simulink model "Overtaking"  (R2024a)
settings: Solver=FixedStepDiscrete  StartTime=0.0  StopTime=inf  FixedStep=0.001  RelTol=1e-3  EnableMultiTasking=on
undefined symbols (not defined in the file): route1_frenet, route1_waypoint, route2_frenet, route2_waypoint, route3_frenet, route3_waypoint, route4_frenet, route4_waypoint, route5_frenet, route5_waypoint
libraries: CarMaker4SL x46, simulink x1, slpidlib x1
(part 2 of 3)

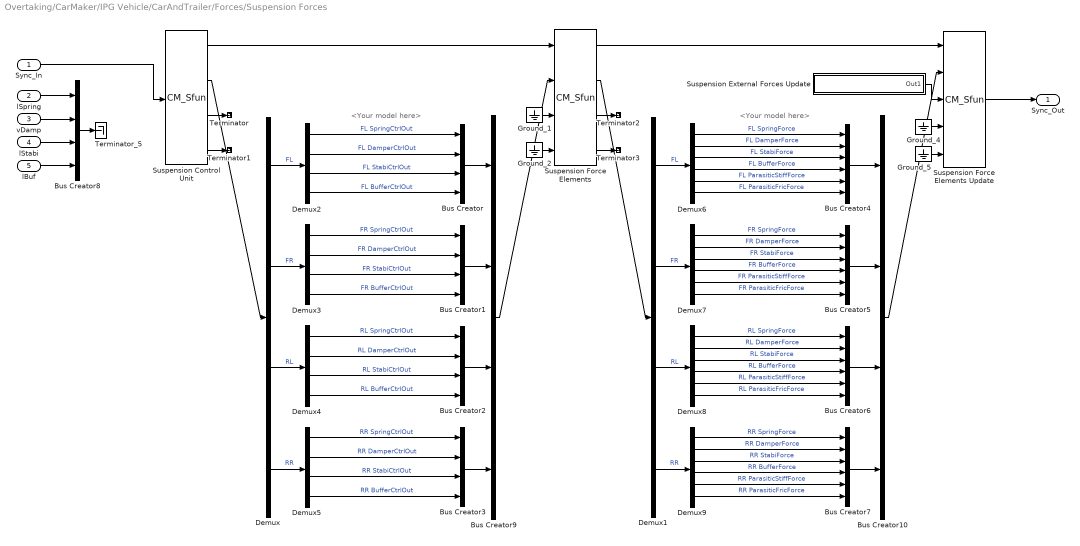
== system Overtaking/CarMaker/IPG Vehicle/CarAndTrailer/Forces/Suspension Forces ==
  note: <Your model here>
  note: <Your model here>
  Sync_In : Inport
  lSpring : Inport  Port=2
  vDamp : Inport  Port=3
  lStabi : Inport  Port=4
  lBuf : Inport  Port=5
  Bus Creator{,1..3,8..10} (7 alike) : BusCreator  Inputs=4
  Bus Creator{4..7} (4 alike) : BusCreator  Inputs=6
  Demux{,1..5} (6 alike) : Demux
  Demux{6..9} (4 alike) : Demux  Outputs=6
  Ground_{1..2,4..5} (4 alike) : Ground
  Suspension Control Unit : S-Function  FunctionName=CM_Sfun  Parameters='ForcesSuspControl'  SFunctionDeploymentMode=off  EnableBusSupport=off
  Suspension External Forces Update : Subsystem
  Suspension Force Elements : S-Function  FunctionName=CM_Sfun  Parameters='ForcesSusp'  SFunctionDeploymentMode=off  EnableBusSupport=off
  Suspension Force Elements Update : S-Function  FunctionName=CM_Sfun  Parameters='ForcesSuspUpd'  SFunctionDeploymentMode=off  EnableBusSupport=off
  Terminator{,1..3} (4 alike) : Terminator
  Terminator_5 : Terminator
  Sync_Out : Outport  VectorParamsAs1DForOutWhenUnconnected=off
  wires:
  vDamp/1 -> Bus Creator8/2
  lStabi/1 -> Bus Creator8/3
  lBuf/1 -> Bus Creator8/4
  lSpring/1 -> Bus Creator8/1
  Bus Creator4/1 -> Bus Creator10/1
  Bus Creator5/1 -> Bus Creator10/2
  Bus Creator6/1 -> Bus Creator10/3
  Bus Creator7/1 -> Bus Creator10/4
  Demux6/1 -> Bus Creator4/1  "FL SpringForce"
  Demux9/1 -> Bus Creator7/1  "RR SpringForce"
  Demux9/2 -> Bus Creator7/2  "RR DamperForce"
  Demux9/3 -> Bus Creator7/3  "RR StabiForce"
  Demux9/4 -> Bus Creator7/4  "RR BufferForce"
  Demux9/5 -> Bus Creator7/5  "RR ParasiticStiffForce"
  Demux9/6 -> Bus Creator7/6  "RR ParasiticFricForce"
  Demux8/1 -> Bus Creator6/1  "RL SpringForce"
  Demux8/2 -> Bus Creator6/2  "RL DamperForce"
  Demux8/4 -> Bus Creator6/4  "RL BufferForce"
  Demux8/5 -> Bus Creator6/5  "RL ParasiticStiffForce"
  Demux8/6 -> Bus Creator6/6  "RL ParasiticFricForce"
  Demux8/3 -> Bus Creator6/3  "RL StabiForce"
  Demux7/1 -> Bus Creator5/1  "FR SpringForce"
  Demux7/2 -> Bus Creator5/2  "FR DamperForce"
  Demux7/3 -> Bus Creator5/3  "FR StabiForce"
  Demux7/4 -> Bus Creator5/4  "FR BufferForce"
  Demux7/5 -> Bus Creator5/5  "FR ParasiticStiffForce"
  Demux7/6 -> Bus Creator5/6  "FR ParasiticFricForce"
  Demux6/2 -> Bus Creator4/2  "FL DamperForce"
  Demux6/3 -> Bus Creator4/3  "FL StabiForce"
  Demux6/4 -> Bus Creator4/4  "FL BufferForce"
  Demux6/5 -> Bus Creator4/5  "FL ParasiticStiffForce"
  Demux6/6 -> Bus Creator4/6  "FL ParasiticFricForce"
  Demux/1 -> Demux2/1  "FL"
  Bus Creator1/1 -> Bus Creator9/2
  Demux/2 -> Demux3/1  "FR"
  Bus Creator2/1 -> Bus Creator9/3
  Demux/3 -> Demux4/1  "RL"
  Bus Creator3/1 -> Bus Creator9/4
  Demux2/1 -> Bus Creator/1  "FL SpringCtrlOut"
  Demux/4 -> Demux5/1  "RR"
  Demux5/1 -> Bus Creator3/1  "RR SpringCtrlOut"
  Demux5/2 -> Bus Creator3/2  "RR DamperCtrlOut"
  Demux5/3 -> Bus Creator3/3  "RR StabiCtrlOut"
  Demux5/4 -> Bus Creator3/4  "RR BufferCtrlOut"
  Demux4/1 -> Bus Creator2/1  "RL SpringCtrlOut"
  Demux4/2 -> Bus Creator2/2  "RL DamperCtrlOut"
  Demux4/4 -> Bus Creator2/4  "RL BufferCtrlOut"
  Demux4/3 -> Bus Creator2/3  "RL StabiCtrlOut"
  Demux3/1 -> Bus Creator1/1  "FR SpringCtrlOut"
  Demux3/2 -> Bus Creator1/2  "FR DamperCtrlOut"
  Demux3/3 -> Bus Creator1/3  "FR StabiCtrlOut"
  Demux3/4 -> Bus Creator1/4  "FR BufferCtrlOut"
  Demux2/2 -> Bus Creator/2  "FL DamperCtrlOut"
  Demux2/3 -> Bus Creator/3  "FL StabiCtrlOut"
  Demux2/4 -> Bus Creator/4  "FL BufferCtrlOut"
  Bus Creator/1 -> Bus Creator9/1
  Demux1/1 -> Demux6/1  "FL"
  Demux1/2 -> Demux7/1  "FR"
  Demux1/3 -> Demux8/1  "RL"
  Demux1/4 -> Demux9/1  "RR"
  Suspension Control Unit/2 -> Demux/1
  Suspension Control Unit/3 -> Terminator/1
  Suspension Control Unit/4 -> Terminator1/1
  Sync_In/1 -> Suspension Control Unit/1
  Suspension Force Elements/2 -> Demux1/1
  Suspension Force Elements/3 -> Terminator2/1
  Suspension Force Elements/4 -> Terminator3/1
  Suspension Control Unit/1 -> Suspension Force Elements/1
  Bus Creator9/1 -> Suspension Force Elements/2
  Bus Creator8/1 -> Terminator_5/1
  Ground_1/1 -> Suspension Force Elements/3
  Ground_2/1 -> Suspension Force Elements/4
  Suspension Force Elements Update/1 -> Sync_Out/1
  Suspension Force Elements/1 -> Suspension Force Elements Update/1
  Bus Creator10/1 -> Suspension Force Elements Update/2
  Ground_4/1 -> Suspension Force Elements Update/4
  Ground_5/1 -> Suspension Force Elements Update/5
  Suspension External Forces Update/1(Out1) -> Suspension Force Elements Update/3

== system Overtaking/CarMaker/IPG Vehicle/CarAndTrailer/Forces/Tires ==
  note: The TireXX_Out signals will only be used if FileIdent is "CarMaker-Tire-CM4SL" in the tire parameter file!
      | An example parameter file can be found in Data/Tire/DT_CM4SL_UserTire.
  Sync_In : Inport
  TireFL_In : Inport  Port=2
  TireFR_In : Inport  Port=3
  TireRL_In : Inport  Port=4
  TireRR_In : Inport  Port=5
  Bus Creator{1..4} (4 alike) : BusCreator  Inputs=11
  Demux{1..3,8} (4 alike) : Demux  Outputs=7
      settings: DisplayOption=none
  TireFL : Subsystem
  TireFR : Subsystem
  TireRL : Subsystem
  TireRR : Subsystem
  TireFL_Out : Outport  VectorParamsAs1DForOutWhenUnconnected=off
  TireFR_Out : Outport  Port=2  VectorParamsAs1DForOutWhenUnconnected=off
  TireRL_Out : Outport  Port=3  VectorParamsAs1DForOutWhenUnconnected=off
  TireRR_Out : Outport  Port=4  VectorParamsAs1DForOutWhenUnconnected=off
  wires:
  Sync_In/1 -> TireRR/1(Sync_In), TireRL/1(Sync_In), TireFR/1(Sync_In), TireFL/1(Sync_In)
  Bus Creator4/1 -> TireRR_Out/1
  Bus Creator2/1 -> TireRL_Out/1
  Bus Creator1/1 -> TireFR_Out/1
  Demux3/5 -> TireRR/6(Rim_turnv)  "Tire_In Rim_turnv"
  Demux3/4 -> TireRR/5(Rim_rotv)  "Tire_In Rim_rotv"
  Demux3/1 -> TireRR/2(Load)  "Tire_In Load"
  Demux3/7 -> TireRR/8(muRoad)  "Tire_In mu"
  Demux3/6 -> TireRR/7(InclinAngle)  "Tire_In Camber"
  Demux3/2 -> TireRR/3(vxtrans)  "Tire_In vxtrans"
  Demux3/3 -> TireRR/4(vytrans)  "Tire_In vytrans"
  TireRR/11(AlignTrq) -> Bus Creator4/11  "Tire_Out AlignTrq"
  TireRR/10(RollResist) -> Bus Creator4/10  "Tire_Out RollResist"
  TireRR/9(OverturnTrq) -> Bus Creator4/9  "Tire_Out OverturnTrq"
  TireRR/8(LoadFrc) -> Bus Creator4/8  "Tire_Out LoadFrc"
  TireRR/7(SideFrc) -> Bus Creator4/7  "Tire_Out SideFrc"
  TireRR/6(LongFrc) -> Bus Creator4/6  "Tire_Out LongFrc"
  TireRR/5(vBelt) -> Bus Creator4/5  "Tire_Out vBelt"
  TireRR/4(rBelt_eff) -> Bus Creator4/4  "Tire_Out rBelt_eff"
  TireRR/3(TurnSlp) -> Bus Creator4/3  "Tire_Out TurnSlp"
  TireRR/1(Slp) -> Bus Creator4/1  "Tire_Out Slp"
  TireRR/2(Alpha) -> Bus Creator4/2  "Tire_Out Alpha"
  Demux2/5 -> TireRL/6(Rim_turnv)  "Tire_In Rim_turnv"
  Demux2/4 -> TireRL/5(Rim_rotv)  "Tire_In Rim_rotv"
  Demux2/1 -> TireRL/2(Load)  "Tire_In Load"
  Demux2/7 -> TireRL/8(muRoad)  "Tire_In mu"
  Demux2/6 -> TireRL/7(InclinAngle)  "Tire_In Camber"
  Demux2/2 -> TireRL/3(vxtrans)  "Tire_In vxtrans"
  Demux2/3 -> TireRL/4(vytrans)  "Tire_In vytrans"
  TireRL/11(AlignTrq) -> Bus Creator2/11  "Tire_Out AlignTrq"
  TireRL/10(RollResist) -> Bus Creator2/10  "Tire_Out RollResist"
  TireRL/9(OverturnTrq) -> Bus Creator2/9  "Tire_Out OverturnTrq"
  TireRL/8(LoadFrc) -> Bus Creator2/8  "Tire_Out LoadFrc"
  TireRL/7(SideFrc) -> Bus Creator2/7  "Tire_Out SideFrc"
  TireRL/6(LongFrc) -> Bus Creator2/6  "Tire_Out LongFrc"
  TireRL/5(vBelt) -> Bus Creator2/5  "Tire_Out vBelt"
  TireRL/4(rBelt_eff) -> Bus Creator2/4  "Tire_Out rBelt_eff"
  TireRL/3(TurnSlp) -> Bus Creator2/3  "Tire_Out TurnSlp"
  TireRL/1(Slp) -> Bus Creator2/1  "Tire_Out Slp"
  TireRL/2(Alpha) -> Bus Creator2/2  "Tire_Out Alpha"
  Demux1/5 -> TireFR/6(Rim_turnv)  "Tire_In Rim_turnv"
  Demux1/4 -> TireFR/5(Rim_rotv)  "Tire_In Rim_rotv"
  Demux1/1 -> TireFR/2(Load)  "Tire_In Load"
  Demux1/7 -> TireFR/8(muRoad)  "Tire_In mu"
  Demux1/6 -> TireFR/7(InclinAngle)  "Tire_In Camber"
  Demux1/2 -> TireFR/3(vxtrans)  "Tire_In vxtrans"
  Demux1/3 -> TireFR/4(vytrans)  "Tire_In vytrans"
  TireFR/11(AlignTrq) -> Bus Creator1/11  "Tire_Out AlignTrq"
  TireFR/10(RollResist) -> Bus Creator1/10  "Tire_Out RollResist"
  TireFR/9(OverturnTrq) -> Bus Creator1/9  "Tire_Out OverturnTrq"
  TireFR/8(LoadFrc) -> Bus Creator1/8  "Tire_Out LoadFrc"
  TireFR/7(SideFrc) -> Bus Creator1/7  "Tire_Out SideFrc"
  TireFR/6(LongFrc) -> Bus Creator1/6  "Tire_Out LongFrc"
  TireFR/5(vBelt) -> Bus Creator1/5  "Tire_Out vBelt"
  TireFR/4(rBelt_eff) -> Bus Creator1/4  "Tire_Out rBelt_eff"
  TireFR/3(TurnSlp) -> Bus Creator1/3  "Tire_Out TurnSlp"
  TireFR/1(Slp) -> Bus Creator1/1  "Tire_Out Slp"
  TireFR/2(Alpha) -> Bus Creator1/2  "Tire_Out Alpha"
  Demux8/5 -> TireFL/6(Rim_turnv)  "Tire_In Rim_turnv"
  Demux8/4 -> TireFL/5(Rim_rotv)  "Tire_In Rim_rotv"
  TireFL_In/1 -> Demux8/1
  Demux8/1 -> TireFL/2(Load)  "Tire_In Load"
  Demux8/7 -> TireFL/8(muRoad)  "Tire_In mu"
  Demux8/6 -> TireFL/7(InclinAngle)  "Tire_In Camber"
  Demux8/2 -> TireFL/3(vxtrans)  "Tire_In vxtrans"
  Demux8/3 -> TireFL/4(vytrans)  "Tire_In vytrans"
  TireFL/11(AlignTrq) -> Bus Creator3/11  "Tire_Out AlignTrq"
  TireFL/10(RollResist) -> Bus Creator3/10  "Tire_Out RollResist"
  TireFL/9(OverturnTrq) -> Bus Creator3/9  "Tire_Out OverturnTrq"
  TireFL/8(LoadFrc) -> Bus Creator3/8  "Tire_Out LoadFrc"
  TireFL/7(SideFrc) -> Bus Creator3/7  "Tire_Out SideFrc"
  TireFL/6(LongFrc) -> Bus Creator3/6  "Tire_Out LongFrc"
  TireFL/5(vBelt) -> Bus Creator3/5  "Tire_Out vBelt"
  TireFL/4(rBelt_eff) -> Bus Creator3/4  "Tire_Out rBelt_eff"
  TireFL/3(TurnSlp) -> Bus Creator3/3  "Tire_Out TurnSlp"
  TireFL/1(Slp) -> Bus Creator3/1  "Tire_Out Slp"
  TireFL/2(Alpha) -> Bus Creator3/2  "Tire_Out Alpha"
  Bus Creator3/1 -> TireFL_Out/1
  TireFR_In/1 -> Demux1/1
  TireRL_In/1 -> Demux2/1
  TireRR_In/1 -> Demux3/1

== system Overtaking/CarMaker/IPG Vehicle/CarAndTrailer/Forces/Vehicle Forces ==
  Sync_In : Inport
  Bus Creator1 : BusCreator  Inputs=12
  Bus Creator8 : BusCreator  Inputs=16
  BusCreator1 : BusCreator  Inputs=4
  BusCreator2 : BusCreator  Inputs=9
  Demux : Demux  Outputs=16
      settings: DisplayOption=none
  Demux1 : Demux  Outputs=12
      settings: DisplayOption=none
  Demux2 : Demux  Outputs=13
      settings: DisplayOption=none
  Forces : S-Function  FunctionName=CM_Sfun  Parameters='Forces'  SFunctionDeploymentMode=off  EnableBusSupport=off
  Terminator : Terminator
  Sync_Out : Outport  VectorParamsAs1DForOutWhenUnconnected=off
  Car.Virtual : Outport  Port=2  VectorParamsAs1DForOutWhenUnconnected=off
  Car.Aero : Outport  Port=3  VectorParamsAs1DForOutWhenUnconnected=off
  Car.Load : Outport  Port=4  VectorParamsAs1DForOutWhenUnconnected=off
  wires:
  BusCreator1/1 -> Terminator/1  "Aero IF (in)"
  Demux2/13 -> BusCreator2/9  "car Aero Trq_1 z"
  Demux2/12 -> BusCreator2/8  "car Aero Trq_1 y"
  Demux2/11 -> BusCreator2/7  "car Aero Trq_1 x"
  Demux2/10 -> BusCreator2/6  "car Aero Frc_1 z"
  Demux2/9 -> BusCreator2/5  "car Aero Frc_1 y"
  Demux2/8 -> BusCreator2/4  "car Aero Frc_1 x"
  Demux2/7 -> BusCreator2/3  "car Aero PoA_1 z"
  Demux2/6 -> BusCreator2/2  "car Aero PoA_1 y"
  Demux2/5 -> BusCreator2/1  "car Aero PoA_1 x"
  Demux2/4 -> BusCreator1/4  "car Aero tau_1"
  Demux2/3 -> BusCreator1/3  "car Aero ApproachVel_1 z"
  Demux2/2 -> BusCreator1/2  "car Aero ApproachVel_1 y"
  Demux2/1 -> BusCreator1/1  "car Aero ApproachVel_1 x"
  Demux/16 -> Bus Creator8/16  "Car Load_3 tz"
  Demux/15 -> Bus Creator8/15  "Car Load_3 ty"
  Demux/14 -> Bus Creator8/14  "Car Load_3 tx"
  Demux/13 -> Bus Creator8/13  "Car Load_3 mass"
  Demux1/12 -> Bus Creator1/12  "Car Virtual Trq_0 z"
  Demux1/11 -> Bus Creator1/11  "Car Virtual Trq_0 y"
  Demux1/10 -> Bus Creator1/10  "Car Virtual Trq_0 x"
  Demux1/9 -> Bus Creator1/9  "Car Virtual Trq_1 z"
  Demux1/8 -> Bus Creator1/8  "Car Virtual Trq_1 y"
  Demux1/7 -> Bus Creator1/7  "Car Virtual Trq_1 x"
  Demux1/6 -> Bus Creator1/6  "Car Virtual Frc_0 z"
  Demux1/5 -> Bus Creator1/5  "Car Virtual Frc_0 y"
  Demux1/4 -> Bus Creator1/4  "Car Virtual Frc_0 x"
  Sync_In/1 -> Forces/1
  Forces/1 -> Sync_Out/1
  BusCreator2/1 -> Car.Aero/1
  Demux1/1 -> Bus Creator1/1  "Car Virtual Frc_1 x"
  Demux1/2 -> Bus Creator1/2  "Car Virtual Frc_1 y"
  Demux1/3 -> Bus Creator1/3  "Car Virtual Frc_1 z"
  Forces/3 -> Demux2/1
  Forces/2 -> Demux1/1
  Bus Creator1/1 -> Car.Virtual/1
  Bus Creator8/1 -> Car.Load/1
  Demux/1 -> Bus Creator8/1  "Car Load_0 mass"
  Demux/2 -> Bus Creator8/2  "Car Load_0 tx"
  Demux/3 -> Bus Creator8/3  "Car Load_0 ty"
  Demux/4 -> Bus Creator8/4  "Car Load_0 tz"
  Demux/5 -> Bus Creator8/5  "Car Load_1 mass"
  Demux/6 -> Bus Creator8/6  "Car Load_1 tx"
  Demux/7 -> Bus Creator8/7  "Car Load_1 ty"
  Demux/8 -> Bus Creator8/8  "Car Load_1 tz"
  Demux/9 -> Bus Creator8/9  "Car Load_2 mass"
  Demux/10 -> Bus Creator8/10  "Car Load_2 tx"
  Demux/11 -> Bus Creator8/11  "Car Load_2 ty"
  Demux/12 -> Bus Creator8/12  "Car Load_2 tz"
  Forces/4 -> Demux/1

== system Overtaking/CarMaker/IPG Vehicle/CarAndTrailer/Trailer/CreateBus Car.Hitch.FrcTrq ==
  In1 : Inport
  Bus Creator7 : BusCreator  Inputs=6
  Demux7 : Demux  Outputs=6
      settings: DisplayOption=none
  Out1 : Outport  VectorParamsAs1DForOutWhenUnconnected=off
  wires:
  In1/1 -> Demux7/1
  Bus Creator7/1 -> Out1/1
  Demux7/6 -> Bus Creator7/6  "Car Hitch Trq2Car z"
  Demux7/5 -> Bus Creator7/5  "Car Hitch Trq2Car y"
  Demux7/4 -> Bus Creator7/4  "Car Hitch Trq2Car x"
  Demux7/3 -> Bus Creator7/3  "Car Hitch Frc2Car z"
  Demux7/2 -> Bus Creator7/2  "Car Hitch Frc2Car y"
  Demux7/1 -> Bus Creator7/1  "Car Hitch Frc2Car x"

== system Overtaking/CarMaker/IPG Vehicle/CarAndTrailer/Trailer/CreateBus Vhcl.Motion ==
  In1 : Inport
  BusCreator : BusCreator  Inputs=15
  Demux : Demux  Outputs=15
      settings: DisplayOption=none
  Out1 : Outport  VectorParamsAs1DForOutWhenUnconnected=off
  wires:
  Demux/15 -> BusCreator/15  "Vhcl YawAcc"
  Demux/14 -> BusCreator/14  "Vhcl YawVel"
  Demux/13 -> BusCreator/13  "Vhcl Yaw"
  Demux/12 -> BusCreator/12  "Vhcl PitchAcc"
  Demux/11 -> BusCreator/11  "Vhcl PitchVel"
  Demux/10 -> BusCreator/10  "Vhcl Pitch"
  Demux/9 -> BusCreator/9  "Vhcl RollAcc"
  Demux/8 -> BusCreator/8  "Vhcl RollVel"
  Demux/7 -> BusCreator/7  "Vhcl Roll"
  Demux/6 -> BusCreator/6  "Vhcl Hitch_Pos z"
  Demux/5 -> BusCreator/5  "Vhcl Hitch_Pos y"
  Demux/4 -> BusCreator/4  "Vhcl Hitch_Pos x"
  Demux/3 -> BusCreator/3  "Vhcl sRoad"
  Demux/2 -> BusCreator/2  "Vhcl Distance"
  Demux/1 -> BusCreator/1  "Vhcl v"
  In1/1 -> Demux/1
  BusCreator/1 -> Out1/1

== system Overtaking/CarMaker/IPG Vehicle/CarAndTrailer/Trailer/CreateBus Vhcl.PoI ==
  In1 : Inport
  Bus Creator3 : BusCreator  Inputs=18
  Demux3 : Demux  Outputs=18
      settings: DisplayOption=none
  Out1 : Outport  VectorParamsAs1DForOutWhenUnconnected=off
  wires:
  Demux3/18 -> Bus Creator3/18  "Vhcl PoI_GCS Elev"
  Demux3/17 -> Bus Creator3/17  "Vhcl PoI_GCS Lat"
  Demux3/16 -> Bus Creator3/16  "Vhcl PoI_GCS Long"
  Demux3/15 -> Bus Creator3/15  "Vhcl PoI_Acc_1 z"
  Demux3/14 -> Bus Creator3/14  "Vhcl PoI_Acc_1 y"
  Demux3/13 -> Bus Creator3/13  "Vhcl PoI_Acc_1 x"
  Demux3/12 -> Bus Creator3/12  "Vhcl PoI_Vel_1 z"
  Demux3/11 -> Bus Creator3/11  "Vhcl PoI_Vel_1 y"
  Demux3/10 -> Bus Creator3/10  "Vhcl PoI_Vel_1 x"
  Demux3/9 -> Bus Creator3/9  "Vhcl PoI_Acc z"
  Demux3/8 -> Bus Creator3/8  "Vhcl PoI_Acc y"
  Demux3/7 -> Bus Creator3/7  "Vhcl PoI_Acc x"
  Demux3/6 -> Bus Creator3/6  "Vhcl PoI_Vel z"
  Demux3/5 -> Bus Creator3/5  "Vhcl PoI_Vel y"
  Demux3/4 -> Bus Creator3/4  "Vhcl PoI_Vel x"
  Demux3/3 -> Bus Creator3/3  "Vhcl PoI_Pos z"
  Demux3/2 -> Bus Creator3/2  "Vhcl PoI_Pos y"
  In1/1 -> Demux3/1
  Bus Creator3/1 -> Out1/1
  Demux3/1 -> Bus Creator3/1  "Vhcl PoI_Pos x"

== system Overtaking/CarMaker/IPG Vehicle/CarAndTrailer/Trailer/CreateBus Vhcl.Steering ==
  In1 : Inport
  Bus Creator3 : BusCreator  Inputs=4
  Demux : Demux
      settings: DisplayOption=none
  Out1 : Outport  VectorParamsAs1DForOutWhenUnconnected=off
  wires:
  Bus Creator3/1 -> Out1/1
  Demux/1 -> Bus Creator3/1  "Vhcl Steering Ang"
  Demux/3 -> Bus Creator3/3  "Vhcl Steering AngAcc"
  Demux/2 -> Bus Creator3/2  "Vhcl Steering AngVel"
  Demux/4 -> Bus Creator3/4  "Vhcl Steering Trq"
  In1/1 -> Demux/1

== system Overtaking/CarMaker/IPG Vehicle/CarAndTrailer/Trailer/CreateBus Vhcl.Wheel.FL ==
  In1 : Inport
  Bus Creator3 : BusCreator  Inputs=14
  Demux3 : Demux  Outputs=14
      settings: DisplayOption=none
  Out1 : Outport  VectorParamsAs1DForOutWhenUnconnected=off
  wires:
  Demux3/14 -> Bus Creator3/14  "Vhcl Wheel FL Trq_WhlBearing"
  Demux3/13 -> Bus Creator3/13  "Vhcl Wheel FL Trq_T2W"
  Demux3/12 -> Bus Creator3/12  "Vhcl Wheel FL SideSlip"
  Demux3/11 -> Bus Creator3/11  "Vhcl Wheel FL LongSlip"
  Demux3/10 -> Bus Creator3/10  "Vhcl Wheel FL vBelt"
  Demux3/9 -> Bus Creator3/9  "Vhcl Wheel FL Fz"
  Demux3/8 -> Bus Creator3/8  "Vhcl Wheel FL Fy"
  Demux3/7 -> Bus Creator3/7  "Vhcl Wheel FL Fx"
  Demux3/6 -> Bus Creator3/6  "Vhcl Wheel FL r_zxy z"
  Demux3/5 -> Bus Creator3/5  "Vhcl Wheel FL r_zxy y"
  Demux3/4 -> Bus Creator3/4  "Vhcl Wheel FL r_zxy x"
  Demux3/3 -> Bus Creator3/3  "Vhcl Wheel FL t z"
  Demux3/2 -> Bus Creator3/2  "Vhcl Wheel FL t y"
  In1/1 -> Demux3/1
  Bus Creator3/1 -> Out1/1
  Demux3/1 -> Bus Creator3/1  "Vhcl Wheel FL t x"

== system Overtaking/CarMaker/IPG Vehicle/CarAndTrailer/Trailer/CreateBus Vhcl.Wheel.FR ==
  In1 : Inport
  Bus Creator3 : BusCreator  Inputs=14
  Demux3 : Demux  Outputs=14
      settings: DisplayOption=none
  Out1 : Outport  VectorParamsAs1DForOutWhenUnconnected=off
  wires:
  Demux3/14 -> Bus Creator3/14  "Vhcl Wheel FR Trq_WhlBearing"
  Demux3/13 -> Bus Creator3/13  "Vhcl Wheel FR Trq_T2W"
  Demux3/12 -> Bus Creator3/12  "Vhcl Wheel FR SideSlip"
  Demux3/11 -> Bus Creator3/11  "Vhcl Wheel FR LongSlip"
  Demux3/10 -> Bus Creator3/10  "Vhcl Wheel FR vBelt"
  Demux3/9 -> Bus Creator3/9  "Vhcl Wheel FR Fz"
  Demux3/8 -> Bus Creator3/8  "Vhcl Wheel FR Fy"
  Demux3/7 -> Bus Creator3/7  "Vhcl Wheel FR Fx"
  Demux3/6 -> Bus Creator3/6  "Vhcl Wheel FR r_zxy z"
  Demux3/5 -> Bus Creator3/5  "Vhcl Wheel FR r_zxy y"
  Demux3/4 -> Bus Creator3/4  "Vhcl Wheel FR r_zxy x"
  Demux3/3 -> Bus Creator3/3  "Vhcl Wheel FR t z"
  Demux3/2 -> Bus Creator3/2  "Vhcl Wheel FR t y"
  In1/1 -> Demux3/1
  Bus Creator3/1 -> Out1/1
  Demux3/1 -> Bus Creator3/1  "Vhcl Wheel FR t x"

== system Overtaking/CarMaker/IPG Vehicle/CarAndTrailer/Trailer/CreateBus Vhcl.Wheel.RL ==
  In1 : Inport
  Bus Creator3 : BusCreator  Inputs=14
  Demux3 : Demux  Outputs=14
      settings: DisplayOption=none
  Out1 : Outport  VectorParamsAs1DForOutWhenUnconnected=off
  wires:
  Demux3/14 -> Bus Creator3/14  "Vhcl Wheel RL Trq_WhlBearing"
  Demux3/13 -> Bus Creator3/13  "Vhcl Wheel RL Trq_T2W"
  Demux3/12 -> Bus Creator3/12  "Vhcl Wheel RL SideSlip"
  Demux3/11 -> Bus Creator3/11  "Vhcl Wheel RL LongSlip"
  Demux3/10 -> Bus Creator3/10  "Vhcl Wheel RL vBelt"
  Demux3/9 -> Bus Creator3/9  "Vhcl Wheel RL Fz"
  Demux3/8 -> Bus Creator3/8  "Vhcl Wheel RL Fy"
  Demux3/7 -> Bus Creator3/7  "Vhcl Wheel RL Fx"
  Demux3/6 -> Bus Creator3/6  "Vhcl Wheel RL r_zxy z"
  Demux3/5 -> Bus Creator3/5  "Vhcl Wheel RL r_zxy y"
  Demux3/4 -> Bus Creator3/4  "Vhcl Wheel RL r_zxy x"
  Demux3/3 -> Bus Creator3/3  "Vhcl Wheel RL t z"
  Demux3/2 -> Bus Creator3/2  "Vhcl Wheel RL t y"
  In1/1 -> Demux3/1
  Bus Creator3/1 -> Out1/1
  Demux3/1 -> Bus Creator3/1  "Vhcl Wheel RL t x"

== system Overtaking/CarMaker/IPG Vehicle/CarAndTrailer/Trailer/CreateBus Vhcl.Wheel.RR ==
  In1 : Inport
  Bus Creator3 : BusCreator  Inputs=14
  Demux3 : Demux  Outputs=14
      settings: DisplayOption=none
  Out1 : Outport  VectorParamsAs1DForOutWhenUnconnected=off
  wires:
  Demux3/14 -> Bus Creator3/14  "Vhcl Wheel RR Trq_WhlBearing"
  Demux3/13 -> Bus Creator3/13  "Vhcl Wheel RR Trq_T2W"
  Demux3/12 -> Bus Creator3/12  "Vhcl Wheel RR SideSlip"
  Demux3/11 -> Bus Creator3/11  "Vhcl Wheel RR LongSlip"
  Demux3/10 -> Bus Creator3/10  "Vhcl Wheel RR vBelt"
  Demux3/9 -> Bus Creator3/9  "Vhcl Wheel RR Fz"
  Demux3/8 -> Bus Creator3/8  "Vhcl Wheel RR Fy"
  Demux3/7 -> Bus Creator3/7  "Vhcl Wheel RR Fx"
  Demux3/6 -> Bus Creator3/6  "Vhcl Wheel RR r_zxy z"
  Demux3/5 -> Bus Creator3/5  "Vhcl Wheel RR r_zxy y"
  Demux3/4 -> Bus Creator3/4  "Vhcl Wheel RR r_zxy x"
  Demux3/3 -> Bus Creator3/3  "Vhcl Wheel RR t z"
  Demux3/2 -> Bus Creator3/2  "Vhcl Wheel RR t y"
  In1/1 -> Demux3/1
  Bus Creator3/1 -> Out1/1
  Demux3/1 -> Bus Creator3/1  "Vhcl Wheel RR t x"

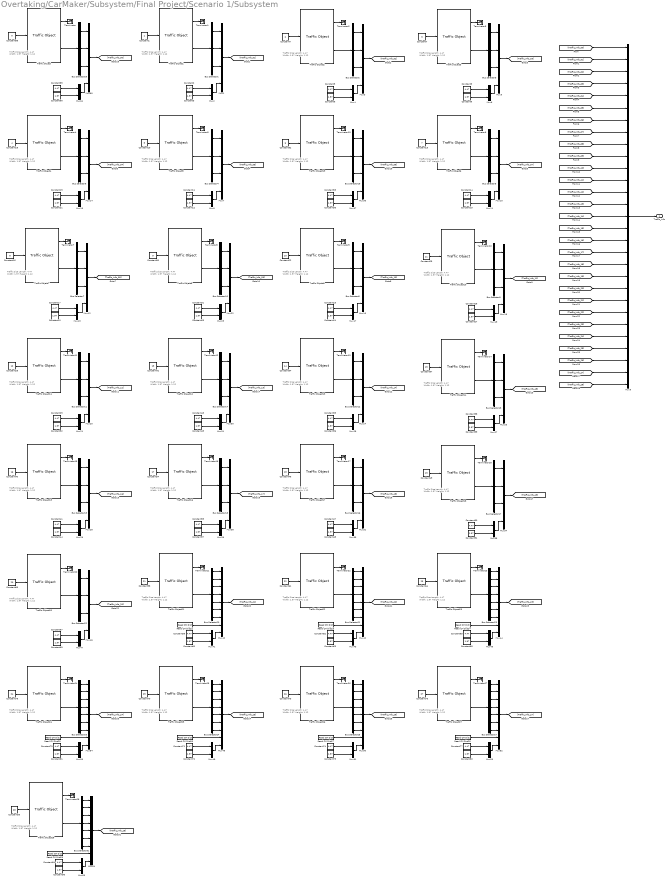
== system Overtaking/CarMaker/Subsystem/Final Project/Scenario 1/Subsystem ==
  note: Traffic Size
      | Length: 4.47
      | Width: 1.97
      | Height: 1.12
  note: Traffic Size
      | Length: 4.47
      | Width: 1.97
      | Height: 1.12
  note: Traffic Size
      | Length: 4.47
      | Width: 1.97
      | Height: 1.12
  note: Traffic Size
      | Length: 4.47
      | Width: 1.97
      | Height: 1.12
  note: Traffic Size
      | Length: 4.47
      | Width: 1.97
      | Height: 1.12
  note: Traffic Size
      | Length: 4.47
      | Width: 1.97
      | Height: 1.12
  note: Traffic Size
      | Length: 4.47
      | Width: 1.97
      | Height: 1.12
  note: Traffic Size
      | Length: 4.47
      | Width: 1.97
      | Height: 1.12
  note: Traffic Size
      | Length: 4.47
      | Width: 1.97
      | Height: 1.12
  note: Traffic Size
      | Length: 4.47
      | Width: 1.97
      | Height: 1.12
  note: Traffic Size
      | Length: 4.47
      | Width: 1.97
      | Height: 1.12
  note: Traffic Size
      | Length: 4.47
      | Width: 1.97
      | Height: 1.12
  note: Traffic Size
      | Length: 4.47
      | Width: 1.97
      | Height: 1.12
  note: Traffic Size
      | Length: 4.47
      | Width: 1.97
      | Height: 1.12
  note: Traffic Size
      | Length: 4.47
      | Width: 1.97
      | Height: 1.12
  note: Traffic Size
      | Length: 4.47
      | Width: 1.97
      | Height: 1.12
  note: Traffic Size
      | Length: 4.47
      | Width: 1.97
      | Height: 1.12
  note: Traffic Size
      | Length: 4.47
      | Width: 1.97
      | Height: 1.12
  note: Traffic Size
      | Length: 4.47
      | Width: 1.97
      | Height: 1.12
  note: Traffic Size
      | Length: 4.47
      | Width: 1.97
      | Height: 1.12
  note: Traffic Size
      | Length: 4.47
      | Width: 1.97
      | Height: 1.12
  note: Traffic Size
      | Length: 4.47
      | Width: 1.97
      | Height: 1.12
  note: Traffic Size
      | Length: 4.47
      | Width: 1.97
      | Height: 1.12
  note: Traffic Size
      | Length: 4.47
      | Width: 1.97
      | Height: 1.12
  note: Traffic Size
      | Length: 4.47
      | Width: 1.97
      | Height: 1.12
  note: Traffic Size
      | Length: 4.47
      | Width: 1.97
      | Height: 1.12
  note: Traffic Size
      | Length: 4.47
      | Width: 1.97
      | Height: 1.12
  note: Traffic Size
      | Length: 4.47
      | Width: 1.97
      | Height: 1.12
  note: Traffic Size
      | Length: 4.47
      | Width: 1.97
      | Height: 1.12
  Bus Selector{1..19,22,29} (21 alike) : BusSelector  OutputSignals=t_0 x,t_0 y,r_zyx z
  Bus Selector{20..21,23..27,31} (8 alike) : BusSelector  OutputSignals=t_0 x,t_0 y,v_0 x,v_0 y,a_0 x,a_0 y,r_zyx z
  Constant1 : Constant
  Constant10 : Constant  Value=5
  Constant{2,5,8,11,14,17,19,23,26,29,31,35,38,41,43,47,50,53,55,59,62,65,67,71,74,77,79,89,94} (29 alike) : Constant  Value=4.47
  Constant{3,6,9,12,15,20..21,24,27,32..33,36,39,44..45,48,51,56..57,60,63,68..69,72,75,80..81,90,96} (29 alike) : Constant  Value=1.97
  Constant13 : Constant  Value=7
  Constant16 : Constant  Value=8
  Constant18 : Constant  Value=4
  Constant22 : Constant  Value=10
  Constant25 : Constant  Value=11
  Constant28 : Constant  Value=12
  Constant30 : Constant  Value=9
  Constant34 : Constant  Value=14
  Constant37 : Constant  Value=15
  Constant4 : Constant  Value=2
  Constant40 : Constant  Value=16
  Constant42 : Constant  Value=13
  Constant46 : Constant  Value=18
  Constant49 : Constant  Value=19
  Constant52 : Constant  Value=6
  Constant54 : Constant  Value=17
  Constant58 : Constant  Value=21
  Constant61 : Constant  Value=22
  Constant64 : Constant  Value=23
  Constant66 : Constant  Value=20
  Constant7 : Constant  Value=3
  Constant70 : Constant  Value=25
  Constant73 : Constant  Value=26
  Constant76 : Constant  Value=27
  Constant78 : Constant  Value=24
  Constant88 : Constant  Value=0
  Constant93 : Constant  Value=28
  Mux{1,3,5,7,10,12,14,16,18,20,22,24,26,28,30,32,34,36,38,46,60} (21 alike) : Mux
  Mux{2,4,6,8,11,13,15,17,19,21,23,25,27,29,31,33,35,37,39,41,43,45,47,49,51,53,55,61,65} (29 alike) : Mux  Inputs=2
  Mux{40,42,44,48,50,52,54,64} (8 alike) : Mux  Inputs=9
  Mux9 : Mux  Inputs=29
  Read CM Dict22 : CarMaker4SL/Read CM Dict  xname=Traffic.T21.rzv  xsync=off  xstime=Inherited
  Read CM Dict23 : CarMaker4SL/Read CM Dict  xname=Traffic.T22.rzv  xsync=off  xstime=Inherited
  Read CM Dict24 : CarMaker4SL/Read CM Dict  xname=Traffic.T23.rzv  xsync=off  xstime=Inherited
  Read CM Dict25 : CarMaker4SL/Read CM Dict  xname=Traffic.T24.rzv  xsync=off  xstime=Inherited
  Read CM Dict26 : CarMaker4SL/Read CM Dict  xname=Traffic.T25.rzv  xsync=off  xstime=Inherited
  Read CM Dict27 : CarMaker4SL/Read CM Dict  xname=Traffic.T26.rzv  xsync=off  xstime=Inherited
  Read CM Dict28 : CarMaker4SL/Read CM Dict  xname=Traffic.T27.rzv  xsync=off  xstime=Inherited
  Read CM Dict29 : CarMaker4SL/Read CM Dict  xname=Traffic.T28.rzv  xsync=off  xstime=Inherited
  Terminator{,1..28} (29 alike) : Terminator
  Traffic Object : CarMaker4SL/Traffic Object  xname=T00  ximode=Traffic Id  xstime=Inherited
      settings: SourceProductName=CarMaker4SL
  Traffic Object1 : CarMaker4SL/Traffic Object  xname=T01  ximode=Traffic Id  xstime=Inherited
      settings: SourceProductName=CarMaker4SL
  Traffic Object10 : CarMaker4SL/Traffic Object  xname=T11  ximode=Traffic Id  xstime=Inherited
      settings: SourceProductName=CarMaker4SL
  Traffic Object11 : CarMaker4SL/Traffic Object  xname=T12  ximode=Traffic Id  xstime=Inherited
      settings: SourceProductName=CarMaker4SL
  Traffic Object12 : CarMaker4SL/Traffic Object  xname=T13  ximode=Traffic Id  xstime=Inherited
      settings: SourceProductName=CarMaker4SL
  Traffic Object13 : CarMaker4SL/Traffic Object  xname=T14  ximode=Traffic Id  xstime=Inherited
      settings: SourceProductName=CarMaker4SL
  Traffic Object14 : CarMaker4SL/Traffic Object  xname=T15  ximode=Traffic Id  xstime=Inherited
      settings: SourceProductName=CarMaker4SL
  Traffic Object15 : CarMaker4SL/Traffic Object  xname=T16  ximode=Traffic Id  xstime=Inherited
      settings: SourceProductName=CarMaker4SL
  Traffic Object16 : CarMaker4SL/Traffic Object  xname=T17  ximode=Traffic Id  xstime=Inherited
      settings: SourceProductName=CarMaker4SL
  Traffic Object17 : CarMaker4SL/Traffic Object  xname=T18  ximode=Traffic Id  xstime=Inherited
      settings: SourceProductName=CarMaker4SL
  Traffic Object18 : CarMaker4SL/Traffic Object  xname=T19  ximode=Traffic Id  xstime=Inherited
      settings: SourceProductName=CarMaker4SL
  Traffic Object19 : CarMaker4SL/Traffic Object  xname=T06  ximode=Traffic Id  xstime=Inherited
      settings: SourceProductName=CarMaker4SL
  Traffic Object2 : CarMaker4SL/Traffic Object  xname=T02  ximode=Traffic Id  xstime=Inherited
      settings: SourceProductName=CarMaker4SL
  Traffic Object20 : CarMaker4SL/Traffic Object  xname=T20  ximode=Traffic Id  xstime=Inherited
      settings: SourceProductName=CarMaker4SL
  Traffic Object21 : CarMaker4SL/Traffic Object  xname=T21  ximode=Traffic Id  xstime=Inherited
      settings: SourceProductName=CarMaker4SL
  Traffic Object22 : CarMaker4SL/Traffic Object  xname=T22  ximode=Traffic Id  xstime=Inherited
      settings: SourceProductName=CarMaker4SL
  Traffic Object23 : CarMaker4SL/Traffic Object  xname=T23  ximode=Traffic Id  xstime=Inherited
      settings: SourceProductName=CarMaker4SL
  Traffic Object24 : CarMaker4SL/Traffic Object  xname=T24  ximode=Traffic Id  xstime=Inherited
      settings: SourceProductName=CarMaker4SL
  Traffic Object25 : CarMaker4SL/Traffic Object  xname=T25  ximode=Traffic Id  xstime=Inherited
      settings: SourceProductName=CarMaker4SL
  Traffic Object26 : CarMaker4SL/Traffic Object  xname=T26  ximode=Traffic Id  xstime=Inherited
      settings: SourceProductName=CarMaker4SL
  Traffic Object27 : CarMaker4SL/Traffic Object  xname=T27  ximode=Traffic Id  xstime=Inherited
      settings: SourceProductName=CarMaker4SL
  Traffic Object28 : CarMaker4SL/Traffic Object  xname=T28  ximode=Traffic Id  xstime=Inherited
      settings: SourceProductName=CarMaker4SL
  Traffic Object3 : CarMaker4SL/Traffic Object  xname=T03  ximode=Traffic Id  xstime=Inherited
      settings: SourceProductName=CarMaker4SL
  Traffic Object4 : CarMaker4SL/Traffic Object  xname=T04  ximode=Traffic Id  xstime=Inherited
      settings: SourceProductName=CarMaker4SL
  Traffic Object5 : CarMaker4SL/Traffic Object  xname=T05  ximode=Traffic Id  xstime=Inherited
      settings: SourceProductName=CarMaker4SL
  Traffic Object6 : CarMaker4SL/Traffic Object  xname=T07  ximode=Traffic Id  xstime=Inherited
      settings: SourceProductName=CarMaker4SL
  Traffic Object7 : CarMaker4SL/Traffic Object  xname=T08  ximode=Traffic Id  xstime=Inherited
      settings: SourceProductName=CarMaker4SL
  Traffic Object8 : CarMaker4SL/Traffic Object  xname=T09  ximode=Traffic Id  xstime=Inherited
      settings: SourceProductName=CarMaker4SL
  Traffic Object9 : CarMaker4SL/Traffic Object  xname=T10  ximode=Traffic Id  xstime=Inherited
      settings: SourceProductName=CarMaker4SL
  Traffic_Info : Outport
  wires:
  Mux61/1 -> Mux60/4
  Mux41/1 -> Mux40/9
  [Traffic_Info_28] -> Mux9/29
  [Traffic_Info_04] -> Mux9/5
  [Traffic_Info_24] -> Mux9/25
  [Traffic_Info_09] -> Mux9/10
  [Traffic_Info_25] -> Mux9/26
  Read CM Dict23/1 -> Mux42/8
  Mux40/1 -> [Traffic_Info_21]
  Read CM Dict24/1 -> Mux44/8
  Constant58/1 -> Traffic Object21/1
  Bus Selector21/7 -> Mux42/7  "<r_zyx z>"
  Bus Selector20/6 -> Mux40/6  "<a_0 y>"
  Bus Selector23/4 -> Mux44/4  "<v_0 y>"
  Traffic Object23/2 -> Bus Selector23/1
  Bus Selector23/7 -> Mux44/7  "<r_zyx z>"
  Bus Selector21/2 -> Mux42/2  "<t_0 y>"
  Constant63/1 -> Mux43/2
  Constant68/1 -> Mux45/2
  Bus Selector25/1 -> Mux50/1  "<t_0 x>"
  Bus Selector10/2 -> Mux22/2  "<t_0 y>"
  Mux28/1 -> [Traffic_Info_16]
  Constant43/1 -> Mux31/1
  Constant81/1 -> Mux55/2
  Bus Selector29/3 -> Mux60/3  "<r_zyx z>"
  Bus Selector16/2 -> Mux32/2  "<t_0 y>"
  Read CM Dict25/1 -> Mux54/8
  Constant21/1 -> Mux15/2
  Bus Selector11/2 -> Mux20/2  "<t_0 y>"
  Mux19/1 -> Mux18/4
  Bus Selector20/7 -> Mux40/7  "<r_zyx z>"
  Bus Selector18/1 -> Mux38/1  "<t_0 x>"
  Traffic Object21/2 -> Bus Selector20/1
  Traffic Object16/2 -> Bus Selector18/1
  Mux31/1 -> Mux30/4
  Mux33/1 -> Mux32/4
  Constant54/1 -> Traffic Object16/1
  [Traffic_Info_11] -> Mux9/12
  Bus Selector31/1 -> Mux64/1  "<t_0 x>"
  Mux26/1 -> [Traffic_Info_15]
  Bus Selector15/1 -> Mux28/1  "<t_0 x>"
  Traffic Object26/2 -> Bus Selector25/1
  Mux35/1 -> Mux34/4
  Constant55/1 -> Mux39/1
  Constant37/1 -> Traffic Object14/1
  Bus Selector17/2 -> Mux34/2  "<t_0 y>"
  Constant11/1 -> Mux8/1
  Constant46/1 -> Traffic Object17/1
  Traffic Object18/2 -> Bus Selector17/1
  Constant50/1 -> Mux35/1
  Bus Selector17/3 -> Mux34/3  "<r_zyx z>"
  Traffic Object/1 -> Terminator/1
  Traffic Object18/1 -> Terminator18/1
  Constant57/1 -> Mux39/2
  Traffic Object17/2 -> Bus Selector16/1
  [Traffic_Info_06] -> Mux9/7
  Traffic Object15/1 -> Terminator15/1
  Mux44/1 -> [Traffic_Info_23]
  Constant14/1 -> Mux11/1
  Bus Selector23/1 -> Mux44/1  "<t_0 x>"
  Bus Selector27/5 -> Mux52/5  "<a_0 x>"
  Constant88/1 -> Traffic Object/1
  Bus Selector26/4 -> Mux54/4  "<v_0 y>"
  Bus Selector24/6 -> Mux48/6  "<a_0 y>"
  Bus Selector25/6 -> Mux50/6  "<a_0 y>"
  Mux48/1 -> [Traffic_Info_25]
  Bus Selector26/5 -> Mux54/5  "<a_0 x>"
  Bus Selector29/1 -> Mux60/1  "<t_0 x>"
  Bus Selector26/1 -> Mux54/1  "<t_0 x>"
  Traffic Object27/1 -> Terminator27/1
  Traffic Object27/2 -> Bus Selector27/1
  Constant52/1 -> Traffic Object19/1
  Bus Selector26/7 -> Mux54/7  "<r_zyx z>"
  Traffic Object13/2 -> Bus Selector12/1
  Constant48/1 -> Mux33/2
  Constant47/1 -> Mux33/1
  Mux23/1 -> Mux22/4
  Traffic Object17/1 -> Terminator17/1
  Bus Selector19/3 -> Mux36/3  "<r_zyx z>"
  Bus Selector23/6 -> Mux44/6  "<a_0 y>"
  Traffic Object20/1 -> Terminator20/1
  Traffic Object1/2 -> Bus Selector1/1
  Constant66/1 -> Traffic Object20/1
  Traffic Object12/1 -> Terminator12/1
  Constant76/1 -> Traffic Object27/1
  Traffic Object10/1 -> Terminator10/1
  Bus Selector22/1 -> Mux46/1  "<t_0 x>"
  [Traffic_Info_20] -> Mux9/21
  Constant75/1 -> Mux51/2
  Mux47/1 -> Mux46/4
  Bus Selector26/3 -> Mux54/3  "<v_0 x>"
  Mux29/1 -> Mux28/4
  [Traffic_Info_13] -> Mux9/14
  Bus Selector6/2 -> Mux14/2  "<t_0 y>"
  Constant18/1 -> Traffic Object4/1
  Constant12/1 -> Mux8/2
  Constant1/1 -> Traffic Object1/1
  Bus Selector6/1 -> Mux14/1  "<t_0 x>"
  Bus Selector3/1 -> Mux5/1  "<t_0 x>"
  Mux5/1 -> [Traffic_Info_03]
  Bus Selector31/5 -> Mux64/5  "<a_0 x>"
  Bus Selector3/3 -> Mux5/3  "<r_zyx z>"
  Bus Selector27/6 -> Mux52/6  "<a_0 y>"
  Constant4/1 -> Traffic Object2/1
  Constant6/1 -> Mux4/2
  Bus Selector27/7 -> Mux52/7  "<r_zyx z>"
  Traffic Object2/1 -> Terminator2/1
  Bus Selector2/1 -> Mux3/1  "<t_0 x>"
  Bus Selector21/5 -> Mux42/5  "<a_0 x>"
  [Traffic_Info_14] -> Mux9/15
  Bus Selector20/3 -> Mux40/3  "<v_0 x>"
  Mux2/1 -> Mux1/4
  Bus Selector2/2 -> Mux3/2  "<t_0 y>"
  Constant3/1 -> Mux2/2
  Bus Selector21/4 -> Mux42/4  "<v_0 y>"
  Traffic Object14/2 -> Bus Selector13/1
  Traffic Object28/2 -> Bus Selector31/1
  Mux64/1 -> [Traffic_Info_28]
  Bus Selector31/2 -> Mux64/2  "<t_0 y>"
  Bus Selector23/3 -> Mux44/3  "<v_0 x>"
  Constant74/1 -> Mux51/1
  Read CM Dict27/1 -> Mux50/8
  Traffic Object28/1 -> Terminator28/1
  Traffic Object25/1 -> Terminator25/1
  Traffic Object24/2 -> Bus Selector26/1
  Bus Selector21/1 -> Mux42/1  "<t_0 x>"
  Bus Selector24/1 -> Mux48/1  "<t_0 x>"
  Read CM Dict26/1 -> Mux48/8
  Bus Selector24/3 -> Mux48/3  "<v_0 x>"
  Mux54/1 -> [Traffic_Info_24]
  Constant70/1 -> Traffic Object25/1
  Bus Selector25/7 -> Mux50/7  "<r_zyx z>"
  [Traffic_Info_26] -> Mux9/27
  Mux49/1 -> Mux48/9
  Constant38/1 -> Mux27/1
  Traffic Object23/1 -> Terminator23/1
  Traffic Object14/1 -> Terminator14/1
  Constant45/1 -> Mux31/2
  [Traffic_Info_00] -> Mux9/1
  Traffic Object7/1 -> Terminator7/1
  Constant44/1 -> Mux29/2
  Bus Selector12/3 -> Mux24/3  "<r_zyx z>"
  Bus Selector27/4 -> Mux52/4  "<v_0 y>"
  Mux38/1 -> [Traffic_Info_17]
  [Traffic_Info_01] -> Mux9/2
  Bus Selector23/2 -> Mux44/2  "<t_0 y>"
  Mux50/1 -> [Traffic_Info_26]
  Constant35/1 -> Mux25/1
  Constant28/1 -> Traffic Object11/1
  Constant40/1 -> Traffic Object15/1
  Constant41/1 -> Mux29/1
  Mux53/1 -> Mux52/9
  Mux11/1 -> Mux10/4
  [Traffic_Info_21] -> Mux9/22
  Read CM Dict22/1 -> Mux40/8
  Constant42/1 -> Traffic Object12/1
  Constant34/1 -> Traffic Object13/1
  Constant39/1 -> Mux27/2
  [Traffic_Info_07] -> Mux9/8
  Mux4/1 -> Mux3/4
  Bus Selector10/3 -> Mux22/3  "<r_zyx z>"
  Bus Selector20/2 -> Mux40/2  "<t_0 y>"
  Mux9/1 -> Traffic_Info/1
  Traffic Object26/1 -> Terminator26/1
  Mux3/1 -> [Traffic_Info_02]
  Bus Selector12/2 -> Mux24/2  "<t_0 y>"
  [Traffic_Info_15] -> Mux9/16
  Traffic Object6/2 -> Bus Selector5/1
  Constant8/1 -> Mux6/1
  Constant80/1 -> Mux53/2
  Bus Selector20/5 -> Mux40/5  "<a_0 x>"
  Traffic Object25/2 -> Bus Selector24/1
  [Traffic_Info_03] -> Mux9/4
  Bus Selector9/3 -> Mux18/3  "<r_zyx z>"
  Traffic Object13/1 -> Terminator13/1
  Bus Selector14/3 -> Mux30/3  "<r_zyx z>"
  [Traffic_Info_10] -> Mux9/11
  Mux30/1 -> [Traffic_Info_13]
  Bus Selector15/2 -> Mux28/2  "<t_0 y>"
  Constant26/1 -> Mux19/1
  Constant2/1 -> Mux2/1
  Constant71/1 -> Mux49/1
  Constant25/1 -> Traffic Object10/1
  [Traffic_Info_18] -> Mux9/19
  Mux20/1 -> [Traffic_Info_12]
  Mux51/1 -> Mux50/9
  Constant10/1 -> Traffic Object5/1
  Bus Selector27/1 -> Mux52/1  "<t_0 x>"
  Traffic Object10/2 -> Bus Selector9/1
  Bus Selector31/7 -> Mux64/7  "<r_zyx z>"
  Bus Selector21/3 -> Mux42/3  "<v_0 x>"
  Constant61/1 -> Traffic Object22/1
  Bus Selector11/1 -> Mux20/1  "<t_0 x>"
  [Traffic_Info_05] -> Mux9/6
  [Traffic_Info_27] -> Mux9/28
  Bus Selector31/6 -> Mux64/6  "<a_0 y>"
  Traffic Object3/1 -> Terminator3/1
  Bus Selector4/1 -> Mux7/1  "<t_0 x>"
  Bus Selector11/3 -> Mux20/3  "<r_zyx z>"
  Bus Selector8/3 -> Mux16/3  "<r_zyx z>"
  Constant72/1 -> Mux49/2
  Constant7/1 -> Traffic Object3/1
  Traffic Object11/1 -> Terminator11/1
  Constant65/1 -> Mux45/1
  Mux46/1 -> [Traffic_Info_20]
  Bus Selector21/6 -> Mux42/6  "<a_0 y>"
  Mux21/1 -> Mux20/4
  Mux65/1 -> Mux64/9
  Bus Selector4/2 -> Mux7/2  "<t_0 y>"
  Traffic Object9/2 -> Bus Selector8/1
  [Traffic_Info_12] -> Mux9/13
  Constant64/1 -> Traffic Object23/1
  Constant31/1 -> Mux23/1
  Traffic Object24/1 -> Terminator24/1
  Mux10/1 -> [Traffic_Info_07]
  Traffic Object2/2 -> Bus Selector2/1
  Constant29/1 -> Mux21/1
  Constant23/1 -> Mux17/1
  Bus Selector2/3 -> Mux3/3  "<r_zyx z>"
  Bus Selector24/7 -> Mux48/7  "<r_zyx z>"
  Constant51/1 -> Mux35/2
  Traffic Object/2 -> Bus Selector29/1
  Traffic Object8/2 -> Bus Selector10/1
  Mux13/1 -> Mux12/4
  Bus Selector1/1 -> Mux1/1  "<t_0 x>"
  Read CM Dict28/1 -> Mux52/8
  Bus Selector24/2 -> Mux48/2  "<t_0 y>"
  Mux1/1 -> [Traffic_Info_01]
  Constant89/1 -> Mux61/1
  Bus Selector25/4 -> Mux50/4  "<v_0 y>"
  Bus Selector27/2 -> Mux52/2  "<t_0 y>"
  Traffic Object11/2 -> Bus Selector11/1
  Constant33/1 -> Mux23/2
  Traffic Object8/1 -> Terminator8/1
  Bus Selector7/1 -> Mux12/1  "<t_0 x>"
  Bus Selector10/1 -> Mux22/1  "<t_0 x>"
  Constant22/1 -> Traffic Object9/1
  Traffic Object12/2 -> Bus Selector14/1
  Read CM Dict29/1 -> Mux64/8
  Bus Selector5/1 -> Mux10/1  "<t_0 x>"
  Constant36/1 -> Mux25/2
  Bus Selector23/5 -> Mux44/5  "<a_0 x>"
  Mux25/1 -> Mux24/4
  Bus Selector7/2 -> Mux12/2  "<t_0 y>"
  Mux43/1 -> Mux42/9
  Bus Selector25/3 -> Mux50/3  "<v_0 x>"
  Bus Selector5/3 -> Mux10/3  "<r_zyx z>"
  Traffic Object5/2 -> Bus Selector4/1
  Mux17/1 -> Mux16/4
  Constant13/1 -> Traffic Object6/1
  Constant60/1 -> Mux41/2
  Constant90/1 -> Mux61/2
  Mux55/1 -> Mux54/9
  Mux14/1 -> [Traffic_Info_04]
  [Traffic_Info_23] -> Mux9/24
  Traffic Object6/1 -> Terminator6/1
  Constant62/1 -> Mux43/1
  Constant15/1 -> Mux11/2
  Bus Selector24/5 -> Mux48/5  "<a_0 x>"
  Bus Selector6/3 -> Mux14/3  "<r_zyx z>"
  Mux12/1 -> [Traffic_Info_08]
  Traffic Object5/1 -> Terminator5/1
  [Traffic_Info_08] -> Mux9/9
  Mux7/1 -> [Traffic_Info_05]
  Bus Selector25/2 -> Mux50/2  "<t_0 y>"
  Bus Selector13/3 -> Mux26/3  "<r_zyx z>"
  Bus Selector4/3 -> Mux7/3  "<r_zyx z>"
  Bus Selector16/1 -> Mux32/1  "<t_0 x>"
  Traffic Object7/2 -> Bus Selector7/1
  Constant5/1 -> Mux4/1
  Bus Selector13/1 -> Mux26/1  "<t_0 x>"
  Mux15/1 -> Mux14/4
  Traffic Object4/2 -> Bus Selector6/1
  Mux36/1 -> [Traffic_Info_06]
  [Traffic_Info_16] -> Mux9/17
  Bus Selector18/2 -> Mux38/2  "<t_0 y>"
  Constant24/1 -> Mux17/2
  Constant19/1 -> Mux15/1
  Mux37/1 -> Mux36/4
  Constant16/1 -> Traffic Object7/1
  [Traffic_Info_17] -> Mux9/18
  Traffic Object22/2 -> Bus Selector21/1
  Constant49/1 -> Traffic Object18/1
  Bus Selector18/3 -> Mux38/3  "<r_zyx z>"
  Mux39/1 -> Mux38/4
  Constant53/1 -> Mux37/1
  Mux16/1 -> [Traffic_Info_10]
  Constant94/1 -> Mux65/1
  Constant20/1 -> Mux13/2
  Traffic Object19/1 -> Terminator19/1
  Bus Selector27/3 -> Mux52/3  "<v_0 x>"
  Bus Selector31/3 -> Mux64/3  "<v_0 x>"
  Constant56/1 -> Mux37/2
  Traffic Object3/2 -> Bus Selector3/1
  Traffic Object9/1 -> Terminator9/1
  [Traffic_Info_22] -> Mux9/23
  Bus Selector26/6 -> Mux54/6  "<a_0 y>"
  Bus Selector19/1 -> Mux36/1  "<t_0 x>"
  Bus Selector9/2 -> Mux18/2  "<t_0 y>"
  Traffic Object16/1 -> Terminator16/1
  Bus Selector12/1 -> Mux24/1  "<t_0 x>"
  Bus Selector26/2 -> Mux54/2  "<t_0 y>"
  Bus Selector25/5 -> Mux50/5  "<a_0 x>"
  Constant67/1 -> Mux47/1
  Constant9/1 -> Mux6/2
  Bus Selector16/3 -> Mux32/3  "<r_zyx z>"
  Bus Selector22/2 -> Mux46/2  "<t_0 y>"
  Mux42/1 -> [Traffic_Info_22]
  Mux60/1 -> [Traffic_Info_00]
  Constant17/1 -> Mux13/1
  Constant96/1 -> Mux65/2
  Constant32/1 -> Mux21/2
  Bus Selector14/1 -> Mux30/1  "<t_0 x>"
  Mux8/1 -> Mux7/4
  Bus Selector17/1 -> Mux34/1  "<t_0 x>"
  Bus Selector3/2 -> Mux5/2  "<t_0 y>"
  Traffic Object22/1 -> Terminator22/1
  Bus Selector5/2 -> Mux10/2  "<t_0 y>"
  Bus Selector1/3 -> Mux1/3  "<r_zyx z>"
  Traffic Object4/1 -> Terminator4/1
  Bus Selector15/3 -> Mux28/3  "<r_zyx z>"
  Bus Selector31/4 -> Mux64/4  "<v_0 y>"
  Bus Selector7/3 -> Mux12/3  "<r_zyx z>"
  Constant73/1 -> Traffic Object26/1
  Mux27/1 -> Mux26/4
  Bus Selector8/2 -> Mux16/2  "<t_0 y>"
  Bus Selector1/2 -> Mux1/2  "<t_0 y>"
  Bus Selector22/3 -> Mux46/3  "<r_zyx z>"
  Constant59/1 -> Mux41/1
  [Traffic_Info_02] -> Mux9/3
  Traffic Object15/2 -> Bus Selector15/1
  Mux32/1 -> [Traffic_Info_18]
  Bus Selector9/1 -> Mux18/1  "<t_0 x>"
  Bus Selector13/2 -> Mux26/2  "<t_0 y>"
  Bus Selector19/2 -> Mux36/2  "<t_0 y>"
  Mux18/1 -> [Traffic_Info_11]
  Bus Selector24/4 -> Mux48/4  "<v_0 y>"
  Mux24/1 -> [Traffic_Info_14]
  Constant30/1 -> Traffic Object8/1
  Mux34/1 -> [Traffic_Info_19]
  [Traffic_Info_19] -> Mux9/20
  Bus Selector8/1 -> Mux16/1  "<t_0 x>"
  Bus Selector20/1 -> Mux40/1  "<t_0 x>"
  Mux52/1 -> [Traffic_Info_27]
  Bus Selector14/2 -> Mux30/2  "<t_0 y>"
  Bus Selector29/2 -> Mux60/2  "<t_0 y>"
  Traffic Object21/1 -> Terminator21/1
  Constant77/1 -> Mux53/1
  Constant93/1 -> Traffic Object28/1
  Mux45/1 -> Mux44/9
  Mux22/1 -> [Traffic_Info_09]
  Mux6/1 -> Mux5/4
  Traffic Object19/2 -> Bus Selector19/1
  Constant27/1 -> Mux19/2
  Constant78/1 -> Traffic Object24/1
  Constant69/1 -> Mux47/2
  Constant79/1 -> Mux55/1
  Traffic Object1/1 -> Terminator1/1
  Bus Selector20/4 -> Mux40/4  "<v_0 y>"
  Traffic Object20/2 -> Bus Selector22/1

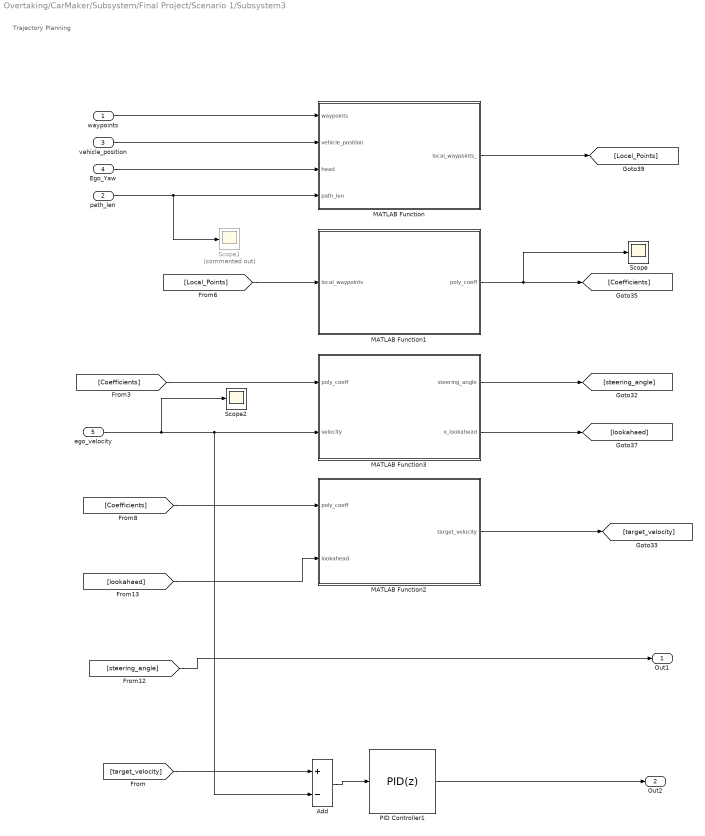
== system Overtaking/CarMaker/Subsystem/Final Project/Scenario 1/Subsystem3 ==
  note: Trajectory Planning
  waypoints : Inport
  path_len : Inport  Port=2
  vehicle_position : Inport  Port=3
  Ego_Yaw : Inport  Port=4
  ego_velocity : Inport  Port=5
  Add : Sum  Inputs=+-
  MATLAB Function : MATLAB Function  TreatAsAtomicUnit=on
  MATLAB Function1 : MATLAB Function  TreatAsAtomicUnit=on
  MATLAB Function2 : MATLAB Function  TreatAsAtomicUnit=on
  MATLAB Function3 : MATLAB Function  TreatAsAtomicUnit=on
  PID Controller1 : slpidlib/PID Controller  Controller=PID  Form=Parallel  TimeDomain=Discrete-time  UseExternalTs=off  SampleTime=-1  IntegratorMethod=Forward Euler  FilterMethod=Forward Euler  ControllerParametersSource=internal  P=3  I=0  UseKiTs=off  D=0.0  UseExternalDerivativeSource=off  N=100  UseFilter=off  TunerSelectOption=Transfer Function Based (PID Tuner App)  InitialConditionSource=internal  InitialConditionForIntegrator=0  InitialConditionForFilter=0  DifferentiatorICPrevScaledInput=0  ExternalReset=none  TrackingMode=off  Kt=1  LimitOutput=off  SatLimitsSource=internal  UpperSaturationLimit=inf  LowerSaturationLimit=-inf  LinearizeAsGain=on  AntiWindupMode=none  Kb=1  LimitIntegrator=off  UpperIntegratorSaturationLimit=inf  LowerIntegratorSaturationLimit=-inf  POutMin=[]  POutMax=[]  IOutMin=[]  IOutMax=[]  DOutMin=[]  DOutMax=[]  NOutMin=[]  NOutMax=[]  SumOutMin=[]  SumOutMax=[]  SaturationOutMin=[]  SaturationOutMax=[]  PParamMin=[]  PParamMax=[]  IParamMin=[]  IParamMax=[]  DParamMin=[]  DParamMax=[]  NParamMin=[]  NParamMax=[]  KbParamMin=[]  KbParamMax=[]  KtParamMin=[]  KtParamMax=[]  KbOutMin=[]  KbOutMax=[]  KtOutMin=[]  KtOutMax=[]  IntegratorOutMin=[]  IntegratorOutMax=[]  FilterOutMin=[]  FilterOutMax=[]  SumI1OutMin=[]  SumI1OutMax=[]  SumI2OutMin=[]  SumI2OutMax=[]  SumI3OutMin=[]  SumI3OutMax=[]  SumI4OutMin=[]  SumI4OutMax=[]  SumDOutMin=[]  SumDOutMax=[]  DifferentiatorOutMin=[]  DifferentiatorOutMax=[]  FilterDiffOutCoefMin=[]  FilterDiffOutCoefMax=[]  ReciprocalOutMin=[]  ReciprocalOutMax=[]  SumDenOutMin=[]  SumDenOutMax=[]  SumNumOutMin=[]  SumNumOutMax=[]  DivideOutMin=[]  DivideOutMax=[]  UdiffTsProdOutMin=[]  UdiffTsProdOutMax=[]  NTsProdOutMin=[]  NTsProdOutMax=[]  UintegralTsProdOutMin=[]  UintegralTsProdOutMax=[]  UngainTsProdOutMin=[]  UngainTsProdOutMax=[]  ClampingZeroOutDataTypeStr=Inherit: Inherit via back propagation  ClampingZeroOutMin=[]  ClampingZeroOutMax=[]  FilterDenConstantOutDataTypeStr=Inherit: Inherit via back propagation  FilterDenConstantOutMin=[]  FilterDenConstantOutMax=[]  PCopyOutDataTypeStr=Inherit: Inherit via back propagation  PCopyOutMin=[]  PCopyOutMax=[]  NCopyOutDataTypeStr=Inherit: Inherit via back propagation  NCopyOutMin=[]  NCopyOutMax=[]  IntegratorContinuousStateAttributes=''  IntegratorStateMustResolveToSignalObject=off  IntegratorRTWStateStorageClass=Auto  FilterContinuousStateAttributes=''  FilterStateMustResolveToSignalObject=off  FilterRTWStateStorageClass=Auto  ParallelPVariant=InternalParameters  IdealPVariant=Disabled  IVariant=InternalParameters  DVariant=InternalParameters  IntegratorVariant=Discrete  SatVariant=Disabled  AWVariant=Passthrough  PCopyVariant=Disabled  TRVariant=Disabled  FdbkBlocksVariant=Forward  IdealPFdbkVariant=Disabled  SatFdbkVariant=Disabled  DerivativeFilterVariant=Differentiator  NVariant=Passthrough  NCopyVariant=Disabled_SignalSpec  FilterICVariant=InternalICsDifferentiator  IntegratorICVariant=InternalICs  ExternalResetVariant=Disabled  TRSumVariant=Passthrough  SumFdbkVariant=Disabled  SumVariant=Sum_PID  TsampFilterVariant=InternalTs  TsampNgainVariant=Passthrough  TsampIntegralVariant=Disabled_SignalSpec  ExternalSaturationOutDataTypeStr=Inherit: Same as second input  DerivativeSourceVariant=ErrorSignal
  Scope : Scope
  Scope1 : Scope  Commented=on
  Scope2 : Scope
  Out1 : Outport
  Out2 : Outport  Port=2
  wires:
  [target_velocity] -> Add/1
  vehicle_position/1 -> MATLAB Function/2(vehicle_position)
  PID Controller1/1 -> Out2/1
  [steering_angle] -> Out1/1
  ego_velocity/1 -> MATLAB Function3/2(velocity), Add/2, Scope2/1
  Ego_Yaw/1 -> MATLAB Function/3(head)
  path_len/1 -> MATLAB Function/4(path_len), Scope1/1
  [lookahaed] -> MATLAB Function2/2(lookahead)
  [Coefficients] -> MATLAB Function2/1(poly_coeff)
  MATLAB Function2/1(target_velocity) -> [target_velocity]
  MATLAB Function1/1(poly_coeff) -> [Coefficients], Scope/1
  [Coefficients] -> MATLAB Function3/1(poly_coeff)
  Add/1 -> PID Controller1/1
  MATLAB Function/1(local_waypoints_) -> [Local_Points]
  MATLAB Function3/1(steering_angle) -> [steering_angle]
  MATLAB Function3/2(x_lookahead) -> [lookahaed]
  waypoints/1 -> MATLAB Function/1(waypoints)
  [Local_Points] -> MATLAB Function1/1(local_waypoints)

== system Overtaking/CarMaker/IPG Vehicle/CarAndTrailer/Forces/Suspension Forces/Suspension External Forces Update ==
  Bus Creator21 : BusCreator  Inputs=6
  Bus Creator22 : BusCreator  Inputs=4
  Bus Creator23 : BusCreator  Inputs=4
  From : From  TagVisibility=global
  Ground{32..39} (8 alike) : Ground
  Out1 : Outport
  wires:
  [D] -> Bus Creator21/4
  Ground36/1 -> Bus Creator22/1
  From/1 -> Bus Creator21/1
  [B] -> Bus Creator21/2
  Ground34/1 -> Bus Creator23/3
  Ground32/1 -> Bus Creator23/1
  [C] -> Bus Creator21/3
  Bus Creator23/1 -> Bus Creator21/5
  Ground33/1 -> Bus Creator23/2
  Bus Creator22/1 -> Bus Creator21/6
  Bus Creator21/1 -> Out1/1
  Ground35/1 -> Bus Creator23/4
  Ground39/1 -> Bus Creator22/4
  Ground38/1 -> Bus Creator22/3
  Ground37/1 -> Bus Creator22/2

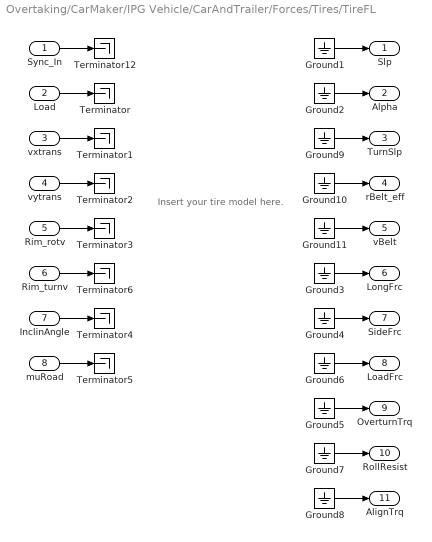
== system Overtaking/CarMaker/IPG Vehicle/CarAndTrailer/Forces/Tires/TireFL ==
  note: Insert your tire model here.
  Sync_In : Inport
  Load : Inport  Port=2
  vxtrans : Inport  Port=3
  vytrans : Inport  Port=4
  Rim_rotv : Inport  Port=5
  Rim_turnv : Inport  Port=6
  InclinAngle : Inport  Port=7
  muRoad : Inport  Port=8
  Ground{1..11} (11 alike) : Ground
  Terminator{,1..6,12} (8 alike) : Terminator
  Slp : Outport  VectorParamsAs1DForOutWhenUnconnected=off
  Alpha : Outport  Port=2  VectorParamsAs1DForOutWhenUnconnected=off
  TurnSlp : Outport  Port=3  VectorParamsAs1DForOutWhenUnconnected=off
  rBelt_eff : Outport  Port=4  VectorParamsAs1DForOutWhenUnconnected=off
  vBelt : Outport  Port=5  VectorParamsAs1DForOutWhenUnconnected=off
  LongFrc : Outport  Port=6  VectorParamsAs1DForOutWhenUnconnected=off
  SideFrc : Outport  Port=7  VectorParamsAs1DForOutWhenUnconnected=off
  LoadFrc : Outport  Port=8  VectorParamsAs1DForOutWhenUnconnected=off
  OverturnTrq : Outport  Port=9  VectorParamsAs1DForOutWhenUnconnected=off
  RollResist : Outport  Port=10  VectorParamsAs1DForOutWhenUnconnected=off
  AlignTrq : Outport  Port=11  VectorParamsAs1DForOutWhenUnconnected=off
  wires:
  Ground11/1 -> vBelt/1
  Ground10/1 -> rBelt_eff/1
  Ground9/1 -> TurnSlp/1
  Rim_turnv/1 -> Terminator6/1
  Sync_In/1 -> Terminator12/1
  Ground2/1 -> Alpha/1
  Ground3/1 -> LongFrc/1
  Ground4/1 -> SideFrc/1
  Ground5/1 -> OverturnTrq/1
  vxtrans/1 -> Terminator1/1
  vytrans/1 -> Terminator2/1
  Rim_rotv/1 -> Terminator3/1
  InclinAngle/1 -> Terminator4/1
  muRoad/1 -> Terminator5/1
  Load/1 -> Terminator/1
  Ground1/1 -> Slp/1
  Ground6/1 -> LoadFrc/1
  Ground7/1 -> RollResist/1
  Ground8/1 -> AlignTrq/1
